simulink model "BuckFeedbackExampleCh9PID"  (Simulink 8.0)
settings: Solver=ode45  StartTime=0.0  StopTime=0.1  MaxStep=1e-6  RelTol=1e-3
settings Model: Creator=rwe  LastModifiedBy=rwe
settings DataIOCC: SignalLoggingSaveFormat=ModelDataLogs
settings DebuggingCC: FcnCallInpInsideContextMsg=UseLocalSettings
settings GRTTargetCC: CombineOutputUpdateFcns=off  GRTInterface=on

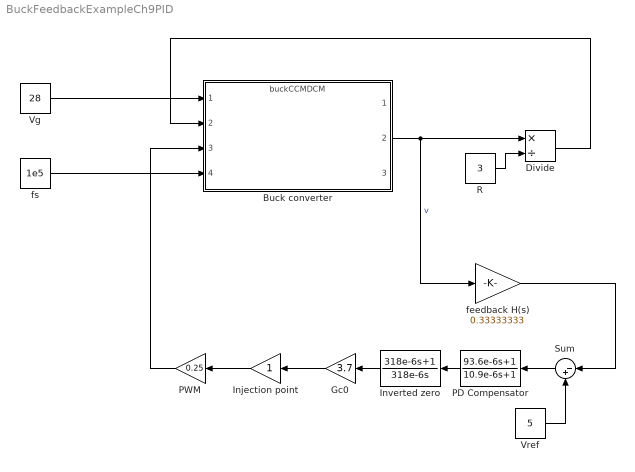
== system BuckFeedbackExampleCh9PID ==
  " Inverted zero" : TransferFcn  Numerator=[318e-6 1]  Denominator=[318e-6 0]
  Buck converter : ModelReference  ModelNameDialog=buckCCMDCM  ModelReferenceVersion=1.29  CopyOfModelName=buckCCMDCM  DefaultDataLogging=off
  Divide : Product  Inputs=*/
  Gc0 : Gain  Gain=3.7
  Injection point : Gain
  PD Compensator : TransferFcn  Numerator=[93.6e-6 1]  Denominator=[10.9e-6 1]
  PWM : Gain  Gain=0.25
  R : Constant  Value=3
  Sum : Sum  Inputs=|-+
  Vg : Constant  Value=28
  Vref : Constant  Value=5
  feedback H(s) : Gain  Gain=0.33333333
  fs : Constant  Value=1e5
  wires:
  Vg/1 -> Buck converter/1
  Buck converter/2 -> Divide/1, feedback H(s)/1  "v"
  Divide/1 -> Buck converter/2
  R/1 -> Divide/2
  fs/1 -> Buck converter/4
  feedback H(s)/1 -> Sum/1
  Vref/1 -> Sum/2
  Sum/1 -> PD Compensator/1
  PWM/1 -> Buck converter/3
  Gc0/1 -> Injection point/1
  Injection point/1 -> PWM/1
  PD Compensator/1 -> " Inverted zero"/1
  " Inverted zero"/1 -> Gc0/1
